simulink model "hw1"  (R2019a)
settings: Solver=VariableStepAuto  StartTime=0.0  StopTime=10.0  MaxStep=0.003  MinStep=0.001  RelTol=1e-3
settings Model: Creator=toshiba1000  LastModifiedBy=toshiba1000
settings SolverCC: InitialStep=0.002

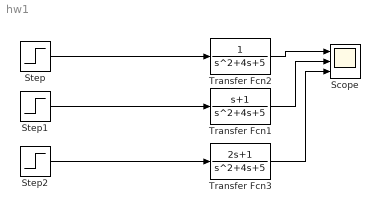
== system hw1 ==
  Scope : Scope  NumInputPorts=3
  Step : Step  SampleTime=0
  Step1 : Step  SampleTime=0
  Step2 : Step  SampleTime=0
  Transfer Fcn1 : TransferFcn  Numerator=[1 1]  Denominator=[1 4 5]
  Transfer Fcn2 : TransferFcn  Denominator=[1 4 5]
  Transfer Fcn3 : TransferFcn  Numerator=[2 1]  Denominator=[1 4 5]
  wires:
  Transfer Fcn2/1 -> Scope/1
  Step/1 -> Transfer Fcn2/1
  Step1/1 -> Transfer Fcn1/1
  Step2/1 -> Transfer Fcn3/1
  Transfer Fcn1/1 -> Scope/2
  Transfer Fcn3/1 -> Scope/3
